simulink model "soc_swhw_fpga"  (R2021a)
settings: Solver=FixedStepAuto  StartTime=0.0  StopTime=10.0  RelTol=1e-3  EnableMultiTasking=on
PreLoadFcn:
  | hsb.blkcb2.defineTypes;
  | sampleTime = 0.1e-6;
values from neighbouring files (symbols this model uses):
  frameSize = 400    [workspace.mat]
  quantizationBits = 8    [workspace.mat]
libraries: hwlogicconnlib x4
settings Model: Creator=The MathWorks, Inc.  LastModifiedBy=AliReza
settings SolverCC: AlgebraicLoopSolver=TrustRegion  PositivePriorityOrder=on
settings DataIOCC: ReturnWorkspaceOutputs=off
settings OptimizationCC: DefaultParameterBehavior=Inlined  EnhancedBackFolding=on  PassReuseOutputArgsAs=Individual arguments  MaxStackSize=64  OptimizeBlockOrder=speed  DifferentSizesBufferReuse=on  OptimizationCustomize=off  EfficientTunableParamExpr=on
settings DebuggingCC: SignalRangeChecking=warning  ParameterTunabilityLossMsg=error  SFMachineParentedDataDiag=warning  ArithmeticOperatorsInVariantConditions=warning
settings HardwareCC: ProdBitPerPointer=32  ProdBitPerSizeT=32  ProdBitPerPtrDiffT=32  ProdLargestAtomicFloat=None  ProdIntDivRoundTo=Undefined  ProdEndianess=Unspecified  ProdWordSize=32  ProdHWDeviceType=ASIC/FPGA->ASIC/FPGA  TargetBitPerPointer=64  TargetBitPerSizeT=64  TargetBitPerPtrDiffT=64  TargetLongLongMode=on  TargetIntDivRoundTo=Zero  TargetEndianess=LittleEndian  TargetWordSize=64  TargetHWDeviceType=Custom Processor->MATLAB Host Computer  ProdEqTarget=off
settings SFSimCC: SimUseLocalCustomCode=off  MATLABDynamicMemAlloc=off
settings RTWCC: SystemTargetFile=ert.tlc  TemplateMakefile=ert_default_tmf  GenerateReport=on  RTWUseLocalCustomCode=off  Toolchain=Linaro AArch32 Linux v6.3.1  IncludeHyperlinkInReport=on  LaunchReport=on  GenerateTraceInfo=on  GenerateTraceReport=on  GenerateTraceReportSl=on  GenerateTraceReportSf=on  GenerateTraceReportEml=on
settings CodeAppCC: ForceParamTrailComments=on  IgnoreCustomStorageClasses=off  OperatorAnnotations=on  SimulinkDataObjDesc=on  SFDataObjDesc=on  InsertBlockDesc=on
settings ERTTargetCC: ERTCustomFileTemplate=example_file_process.tlc

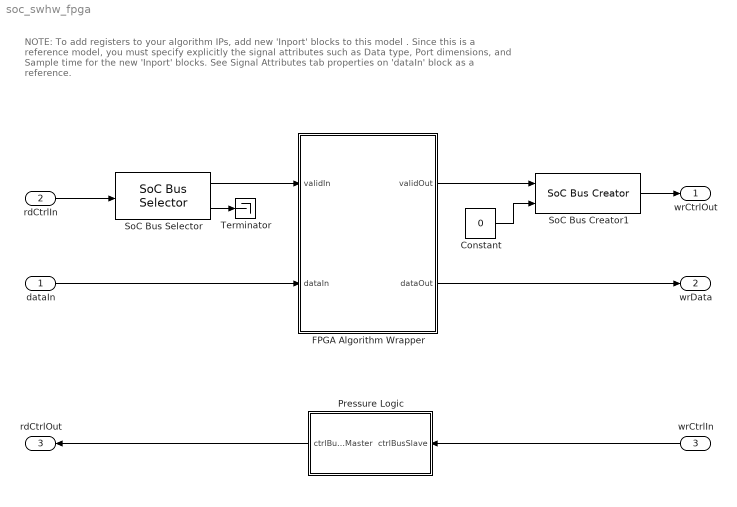
== system soc_swhw_fpga ==
  note: NOTE:
      | To add registers to your algorithm IPs, add new 'Inport' blocks to this model . Since this is a reference model, you must specify explicitly the signal attributes such as Data type, Port dimensions, and Sample time for the new 'Inport' blocks. See Signal Attributes tab properties on 'dataIn' block as a reference.
  dataIn : Inport  OutDataTypeStr=single  SampleTime=sampleTime
  rdCtrlIn : Inport  Port=2  OutDataTypeStr=Bus: StreamM2SBusObj
  wrCtrlIn : Inport  Port=3  OutDataTypeStr=Bus: StreamS2MBusObj
  Constant : Constant  Value=0  OutDataTypeStr=boolean
  FPGA Algorithm Wrapper : Subsystem
  Pressure Logic : Subsystem
  SoC Bus Creator1 : hwlogicconnlib/SoC Bus Creator  Protocol=Data stream  ctrltype=Valid
      settings: SourceProductBaseCode=HW
  SoC Bus Selector : hwlogicconnlib/SoC Bus Selector  Protocol=Data stream  ctrltype=Valid
      settings: SourceProductBaseCode=HW
  Terminator : Terminator
  wrCtrlOut : Outport  OutDataTypeStr=Bus: StreamM2SBusObj  InitialOutput=0
  wrData : Outport  Port=2  InitialOutput=0
  rdCtrlOut : Outport  Port=3  OutDataTypeStr=Bus: StreamS2MBusObj  VectorParamsAs1DForOutWhenUnconnected=off
  wires:
  rdCtrlIn/1 -> SoC Bus Selector/1
  SoC Bus Selector/2 -> Terminator/1
  FPGA Algorithm Wrapper/2(dataOut) -> wrData/1
  Constant/1 -> SoC Bus Creator1/2
  FPGA Algorithm Wrapper/1(validOut) -> SoC Bus Creator1/1
  SoC Bus Creator1/1 -> wrCtrlOut/1
  wrCtrlIn/1 -> Pressure Logic/1(ctrlBusSlave)
  Pressure Logic/1(ctrlBusMaster) -> rdCtrlOut/1
  SoC Bus Selector/1 -> FPGA Algorithm Wrapper/1(validIn)
  dataIn/1 -> FPGA Algorithm Wrapper/2(dataIn)

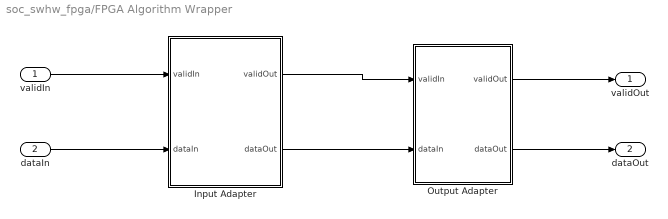
== system soc_swhw_fpga/FPGA Algorithm Wrapper ==
  validIn : Inport
  dataIn : Inport  Port=2
  Input Adapter : Subsystem
  Output Adapter : Subsystem
  validOut : Outport  InitialOutput=0
  dataOut : Outport  Port=2  InitialOutput=0
  wires:
  validIn/1 -> Input Adapter/1(validIn)
  dataIn/1 -> Input Adapter/2(dataIn)
  Input Adapter/1(validOut) -> Output Adapter/1(validIn)
  Input Adapter/2(dataOut) -> Output Adapter/2(dataIn)
  Output Adapter/1(validOut) -> validOut/1
  Output Adapter/2(dataOut) -> dataOut/1

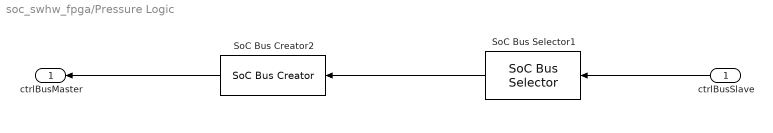
== system soc_swhw_fpga/Pressure Logic ==
  ctrlBusSlave : Inport
  SoC Bus Creator2 : hwlogicconnlib/SoC Bus Creator  Protocol=Data stream  ctrltype=Ready
      settings: SourceProductBaseCode=HW
  SoC Bus Selector1 : hwlogicconnlib/SoC Bus Selector  Protocol=Data stream  ctrltype=Ready
      settings: SourceProductBaseCode=HW
  ctrlBusMaster : Outport
  wires:
  SoC Bus Selector1/1 -> SoC Bus Creator2/1
  SoC Bus Creator2/1 -> ctrlBusMaster/1
  ctrlBusSlave/1 -> SoC Bus Selector1/1

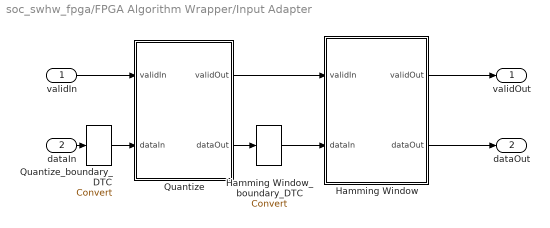
== system soc_swhw_fpga/FPGA Algorithm Wrapper/Input Adapter ==
  validIn : Inport
  dataIn : Inport  Port=2
  Hamming Window : Subsystem
  Hamming Window_boundary_DTC : DataTypeConversion  SaturateOnIntegerOverflow=on  RndMeth=Zero
  Quantize : Subsystem  TreatAsAtomicUnit=on
  Quantize_boundary_DTC : DataTypeConversion  SaturateOnIntegerOverflow=on  RndMeth=Zero
  validOut : Outport
  dataOut : Outport  Port=2
  wires:
  validIn/1 -> Quantize/1(validIn)
  Quantize/1(validOut) -> Hamming Window/1(validIn)
  Hamming Window/1(validOut) -> validOut/1
  Hamming Window/2(dataOut) -> dataOut/1
  dataIn/1 -> Quantize_boundary_DTC/1
  Quantize_boundary_DTC/1 -> Quantize/2(dataIn)
  Quantize/2(dataOut) -> Hamming Window_boundary_DTC/1
  Hamming Window_boundary_DTC/1 -> Hamming Window/2(dataIn)

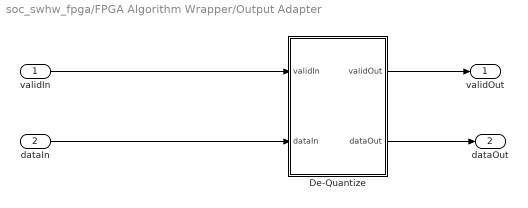
== system soc_swhw_fpga/FPGA Algorithm Wrapper/Output Adapter ==
  validIn : Inport
  dataIn : Inport  Port=2
  De-Quantize : Subsystem  TreatAsAtomicUnit=on
  validOut : Outport
  dataOut : Outport  Port=2
  wires:
  dataIn/1 -> De-Quantize/2(dataIn)
  De-Quantize/2(dataOut) -> dataOut/1
  validIn/1 -> De-Quantize/1(validIn)
  De-Quantize/1(validOut) -> validOut/1

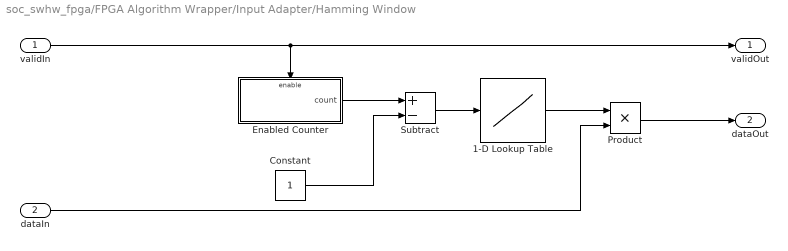
== system soc_swhw_fpga/FPGA Algorithm Wrapper/Input Adapter/Hamming Window ==
  validIn : Inport
  dataIn : Inport  Port=2
  1-D Lookup Table : Lookup_n-D  NumberOfTableDimensions=1  BreakpointsForDimension1=[0:399]  BreakpointsForDimension1FirstPoint=0  IndexSearchMethod=Evenly spaced points  Table=0.54 - (0.46 * cos((2 * pi * (0 : frameSize -1)) / (frameSize - 1)))  TableDataTypeStr=fixdt(0,8,8)  InterpMethod=Flat  RemoveProtectionInput=on  InternalRulePriority=Speed  OutDataTypeStr=fixdt(0,8,8)  RndMeth=Simplest
  Constant : Constant
  Enabled Counter : Subsystem  TreatAsAtomicUnit=on  mask(Counter){maxCount=frameSize}
      mask prompts: maxCount "Maximum count:"
  Product : Product  OutDataTypeStr=int8  RndMeth=Convergent
  Subtract : Sum  Inputs=+-  RndMeth=Simplest
  validOut : Outport  InitialOutput=0
  dataOut : Outport  Port=2  InitialOutput=0
  wires:
  Enabled Counter/1(count) -> Subtract/1
  Constant/1 -> Subtract/2
  Subtract/1 -> 1-D Lookup Table/1
  1-D Lookup Table/1 -> Product/1
  dataIn/1 -> Product/2
  validIn/1 -> validOut/1, Enabled Counter/Enable
  Product/1 -> dataOut/1

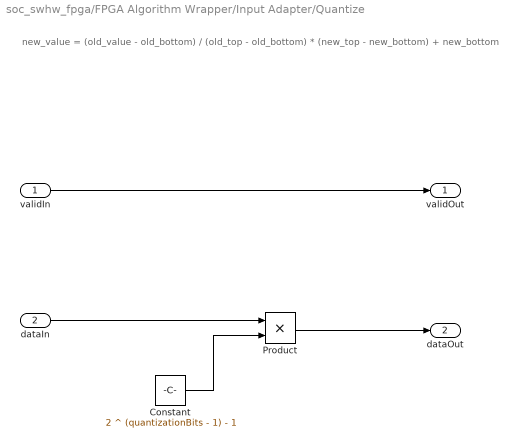
== system soc_swhw_fpga/FPGA Algorithm Wrapper/Input Adapter/Quantize ==
  note: new_value = (old_value - old_bottom) / (old_top - old_bottom) * (new_top - new_bottom) + new_bottom
  validIn : Inport
  dataIn : Inport  Port=2
  Constant : Constant  Value=2 ^ (quantizationBits - 1) - 1  OutDataTypeStr=int8
  Product : Product  OutDataTypeStr=int8  RndMeth=Convergent
  validOut : Outport  InitialOutput=0
  dataOut : Outport  Port=2  InitialOutput=0
  wires:
  dataIn/1 -> Product/1
  validIn/1 -> validOut/1
  Product/1 -> dataOut/1
  Constant/1 -> Product/2

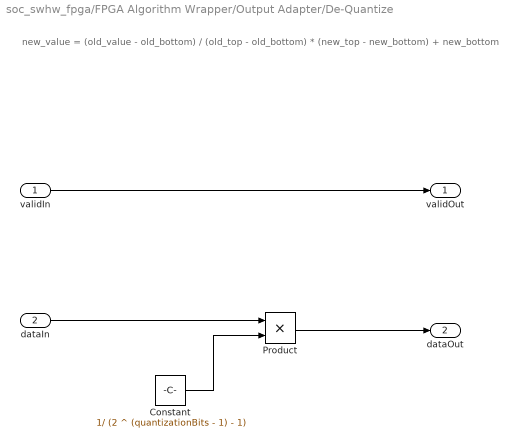
== system soc_swhw_fpga/FPGA Algorithm Wrapper/Output Adapter/De-Quantize ==
  note: new_value = (old_value - old_bottom) / (old_top - old_bottom) * (new_top - new_bottom) + new_bottom
  validIn : Inport
  dataIn : Inport  Port=2
  Constant : Constant  Value=1/ (2 ^ (quantizationBits - 1) - 1)  OutDataTypeStr=fixdt(0,8,8)
  Product : Product  OutDataTypeStr=single  RndMeth=Convergent
  validOut : Outport  InitialOutput=0
  dataOut : Outport  Port=2  InitialOutput=0
  wires:
  dataIn/1 -> Product/1
  validIn/1 -> validOut/1
  Product/1 -> dataOut/1
  Constant/1 -> Product/2

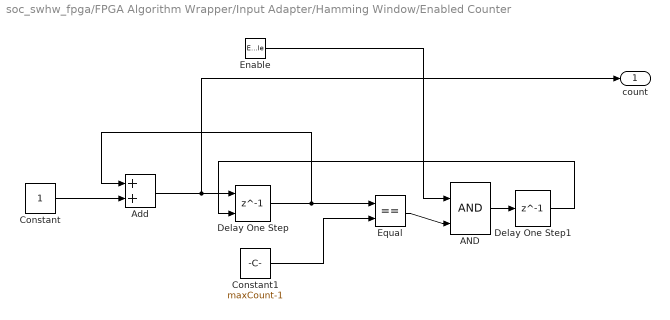
== system soc_swhw_fpga/FPGA Algorithm Wrapper/Input Adapter/Hamming Window/Enabled Counter ==
  Enable : EnablePort  ShowOutputPort=on
  AND : Logic  IconShape=distinctive  AllPortsSameDT=off  OutDataTypeStr=boolean
  Add : Sum  AccumDataTypeStr=uint(floor(log2(maxCount))+1)  OutDataTypeStr=uint(floor(log2(maxCount))+1)  RndMeth=Simplest
  Constant : Constant  OutDataTypeStr=uint(floor(log2(maxCount))+1)
  Constant1 : Constant  Value=maxCount-1  OutDataTypeStr=uint(floor(log2(maxCount))+1)
  Delay One Step : Delay  DelayLength=1  InitialCondition=0  ExternalReset=Rising
      settings: InputPortMap=u0,r5
  Delay One Step1 : Delay  DelayLength=1  InitialCondition=0
  Equal : RelationalOperator  Operator===  OutDataTypeStr=boolean  RndMeth=Simplest
  count : Outport
  wires:
  Constant/1 -> Add/2
  Delay One Step/1 -> Add/1, Equal/1
  Constant1/1 -> Equal/2
  Equal/1 -> AND/2
  Delay One Step1/1 -> Delay One Step/2
  AND/1 -> Delay One Step1/1
  Enable/1 -> AND/1
  Add/1 -> count/1, Delay One Step/1
